simulink model "aileron"  (R2025a)
settings: Solver=VariableStepAuto  StartTime=0.0  StopTime=1.5  RelTol=1e-3
model workspace (MAT data in the model file):
  a1 = 0.5
  a2 = 2
  a3 = 2.5
libraries: simulink x1
settings Model: Creator=JPIRES3  LastModifiedBy=JPIRES3

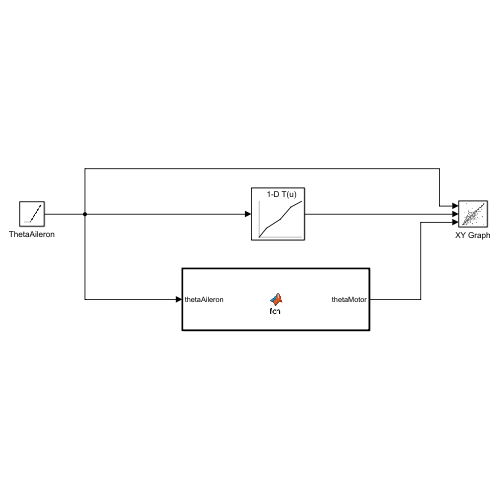
[thumbnail: Simulink's stored preview of the top-level diagram]
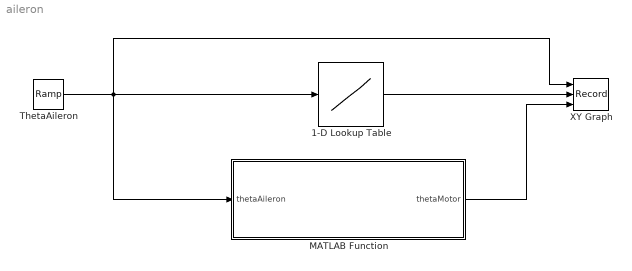
== system aileron ==
  1-D Lookup Table : Lookup_n-D  NumberOfTableDimensions=1  BreakpointsForDimension1=[-pi/4,-pi/6,0,pi/8,pi/4]  Table=[-pi/4,-pi/8,0,pi/6,pi/4]  InternalRulePriority=Speed  RndMeth=Simplest
  MATLAB Function : MATLAB Function  TreatAsAtomicUnit=on
  ThetaAileron : simulink/Sources/Ramp  slope=1  start=0  InitialOutput=-pi/4
  XY Graph : Record  NumPorts=3.0  FileSettingsInternal="{\"entries\":[{\"content\":{\"excelSettings\":{\"content\":{},\"type\":\"Streamout.ExcelSettings\"},\"parquetSettings\":{\"content\":{},\"type\":\"Streamout.ParquetSettings\"}},\"type\":\"Streamout.FileSettingStorage\",\"uuid\":\"\"}],\"packageUris\":[\"http:\\/\\/schema.mathworks.com\\/mf0\\/streamout_blocks\\/R2020a\"],\"version\":\"1.0\"}"  FrameSettings=[0, 0, 0]  Layout=[1 1]  SignalsInternal="{\"entries\":[{\"content\":{\"signals\":[{\"content\":{\"blockPath\":[],\"dimensions\":[1],\"domain\":\"\",\"lineColor\":\"#a2142f\",\"plots\":[ 1 ],\"port\":1,\"sid\":[\"\"],\"signalID\":1,\"signalName\":\"ThetaAileron\"},\"type\":\"RecordBlkView.Signal\",\"uuid\":\"\"},{\"content\":{\"blockPath\":[],\"dimensions\":[1],\"domain\":\"\",\"lineColor\":\"#139fff\",\"plots\":[ 1 ],\"port\":2,\"sid\":[\"\"],\"signalID\":2,\"signalName\":\"1-D Lookup\\nTable\"},\"type\":\"RecordBlkView.Signal\",\"uuid\":\"\"},{\"content\":{\"blockPath\":[],\"dimensions\":[1],\"domain\":\"\",\"lineColor\":\"#ff6929\",\"lineWidth\":2,\"plots\":[ 1 ],\"port\":3,\"sid\":[\"\"],\"signalID\":3,\"signalName\":\"MATLAB Function\"},\"type\":\"RecordBlkView.Signal\",\"uuid\":\"\"}]},\"type\":\"RecordBlkView.InputSignals\",\"uuid\":\"\"}],\"packageUris\":[\"http:\\/\\/schema.mathworks.com\\/mf0\\/streamout_blocks\\/R2020a\"],\"version\":\"1.0\"}"  VisualizationBindings="{\"xyplotplugin\":{\"info\":[{\"series\":[{\"bindingParametersList\":[{\"parameter\":\"X-Axis\",\"signalID\":1,\"signalName\":\"ThetaAileron\"},{\"parameter\":\"Y-Axis\",\"signalID\":2,\"signalName\":\"1-D Lookup\\nTable\"},{\"parameter\":\"X-Axis\",\"signalID\":1,\"signalName\":\"ThetaAileron\"},{\"parameter\":\"Y-Axis\",\"signalID\":2,\"signalName\":\"1-D Lookup\\nTable\"}],\"seriesID\":0},{\"bindingParametersList\":[{\"parameter\":\"X-Axis\",\"signalID\":1,\"signalName\":\"ThetaAileron\"},{\"parameter\":\"Y-Axis\",\"signalID\":3,\"signalName\":\"MATLAB Function\"}],\"seriesID\":1}],\"subplotID\":1}]}}"  CompatibilityTag=XY
  wires:
  ThetaAileron/1 -> 1-D Lookup Table/1, XY Graph/1, MATLAB Function/1(thetaAileron)
  1-D Lookup Table/1 -> XY Graph/2
  MATLAB Function/1(thetaMotor) -> XY Graph/3

== matlab function aileron/MATLAB Function ==
  data: thetaAileron input; thetaMotor output; a3 parameter; a2 parameter; a1 parameter
function thetaMotor = fcn(thetaAileron, a3, a2, a1)

thetaMotor = a1 * thetaAileron * (a2 * thetaAileron^2 + a3 * thetaAileron^4);
